simulink model "signal_conversion_sim"  (R2020b)
settings: Solver=FixedStepAuto  StartTime=0.0  StopTime=simulation_time  RelTol=1e-3
InitFcn:
  | initCallback
StopFcn:
  | stopCallback
values from neighbouring files (symbols this model uses):
  fs = 48e3    (= 48000)    [model_parameters.m]    (also in modelparameters.m)
settings Model: Creator=t96f346  LastModifiedBy=conno
settings DataIOCC: ReturnWorkspaceOutputs=off

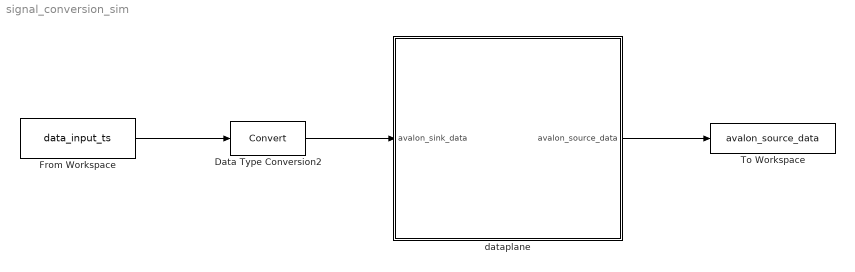
== system signal_conversion_sim ==
  Data Type Conversion2 : DataTypeConversion  RndMeth=Nearest  SaturateOnIntegerOverflow=on
  From Workspace : FromWorkspace  VariableName=data_input_ts  SampleTime=1/fs
  To Workspace : ToWorkspace  VariableName=avalon_source_data  SampleTime=-1
  dataplane : Subsystem  TreatAsAtomicUnit=on
  wires:
  From Workspace/1 -> Data Type Conversion2/1
  Data Type Conversion2/1 -> dataplane/1(avalon_sink_data)
  dataplane/1(avalon_source_data) -> To Workspace/1

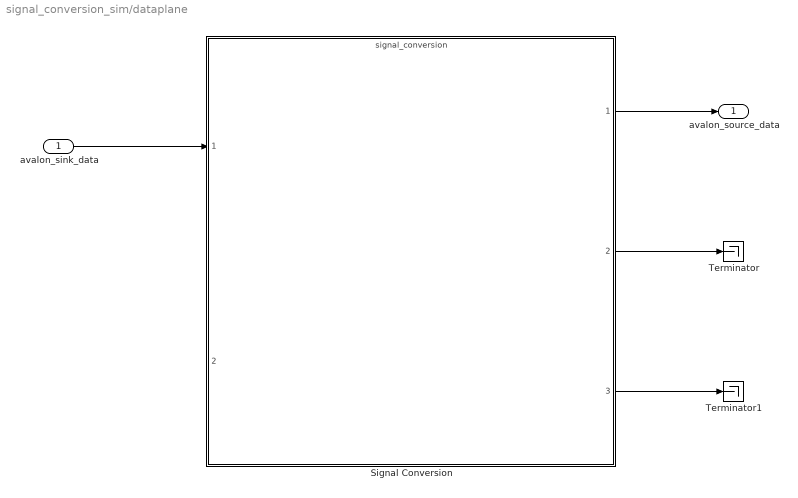
== system signal_conversion_sim/dataplane ==
  avalon_sink_data : Inport  OutDataTypeStr=input_type
  Signal Conversion : ModelReference  ModelNameDialog=signal_conversion.slx  SimulationMode=Normal  ModelReferenceVersion=1.4
  Terminator : Terminator
  Terminator1 : Terminator
  avalon_source_data : Outport  OutDataTypeStr=input_type  VectorParamsAs1DForOutWhenUnconnected=off
  wires:
  avalon_sink_data/1 -> Signal Conversion/1
  Signal Conversion/1 -> avalon_source_data/1
  Signal Conversion/2 -> Terminator/1
  Signal Conversion/3 -> Terminator1/1
